simulink model "three_g"  (R2025a)
settings: Solver=FixedStepDiscrete  StartTime=0.0  StopTime=1  FixedStep=1  RelTol=1e-3
settings Model: Creator=horty  LastModifiedBy=sdarshan
settings DataIOCC: SaveFormat=Array  SignalLogging=off  DSMLogging=off  SaveTime=off  ReturnWorkspaceOutputs=off

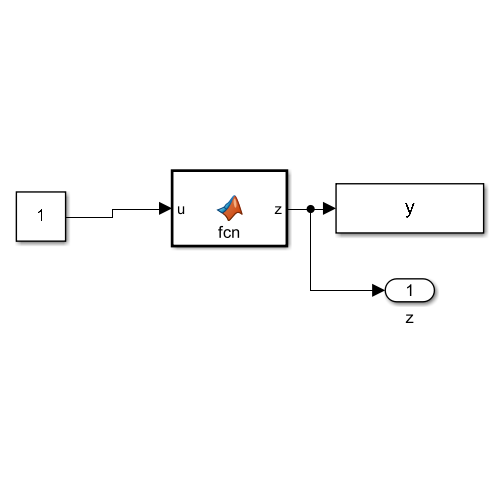
[thumbnail: Simulink's stored preview of the top-level diagram]
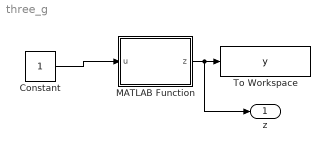
== system three_g ==
  Constant : Constant
  MATLAB Function : MATLAB Function  TreatAsAtomicUnit=on
  To Workspace : ToWorkspace  VariableName=y  SampleTime=-1
      settings: MaxDataPoints=1  Save2DSignal=2-D array (concatenate along first dimension)
  z : Outport
  wires:
  MATLAB Function/1(z) -> z/1, To Workspace/1
  Constant/1 -> MATLAB Function/1(u)

== matlab function three_g/MATLAB Function ==
  data: u input; z output
function z = fcn(u)
%Implement structural analysis code to test if wingbox can sustain -3g
%loads. 
z = u;
